simulink subsystem "Manual_Control_CMDs"  (R2025b)
settings: Solver=VariableStepAuto  StartTime=0.0  StopTime=10.0  RelTol=1e-3
undefined symbols (not defined in the file): EngineThrustCMD
settings Model: Creator=cdriggs  LastModifiedBy=Andrew

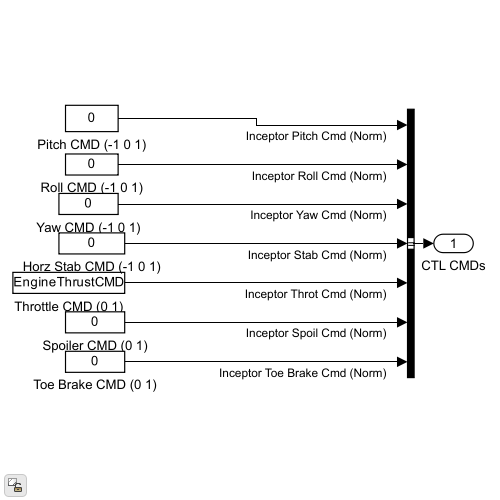
[thumbnail: Simulink's stored preview of the top-level diagram]
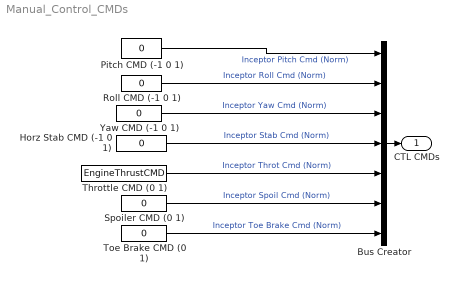
== system Manual_Control_CMDs ==
  Bus Creator : BusCreator  Inputs=7
  Horz Stab CMD (-1 0 1) : Constant  Value=0
  Pitch CMD (-1 0 1) : Constant  Value=0
  Roll CMD (-1 0 1) : Constant  Value=0
  Spoiler CMD (0 1) : Constant  Value=0
  Throttle CMD (0 1) : Constant  Value=EngineThrustCMD
  Toe Brake CMD (0 1) : Constant  Value=0
  Yaw CMD (-1 0 1) : Constant  Value=0
  CTL CMDs : Outport
  wires:
  Pitch CMD (-1 0 1)/1 -> Bus Creator/1  "Inceptor Pitch Cmd (Norm)"
  Roll CMD (-1 0 1)/1 -> Bus Creator/2  "Inceptor Roll Cmd (Norm)"
  Yaw CMD (-1 0 1)/1 -> Bus Creator/3  "Inceptor Yaw Cmd (Norm)"
  Spoiler CMD (0 1)/1 -> Bus Creator/6  "Inceptor Spoil Cmd (Norm)"
  Toe Brake CMD (0 1)/1 -> Bus Creator/7  "Inceptor Toe Brake Cmd (Norm)"
  Horz Stab CMD (-1 0 1)/1 -> Bus Creator/4  "Inceptor Stab Cmd (Norm)"
  Bus Creator/1 -> CTL CMDs/1
  Throttle CMD (0 1)/1 -> Bus Creator/5  "Inceptor Throt Cmd (Norm)"
